simulink model "System"  (R2021b)
settings: Solver=VariableStepAuto  StartTime=0.0  StopTime=10  RelTol=1e-3
values from neighbouring files (symbols this model uses):
  a = 1.2    [new_ref1.mat]
  Cf = 19000    [new_ref1.mat]
  Iz = 3344    [new_ref1.mat]
  m = 2050    [new_ref1.mat]
libraries: simulink x1, mpclib x1
settings Model: Creator=gaura  LastModifiedBy=gaura

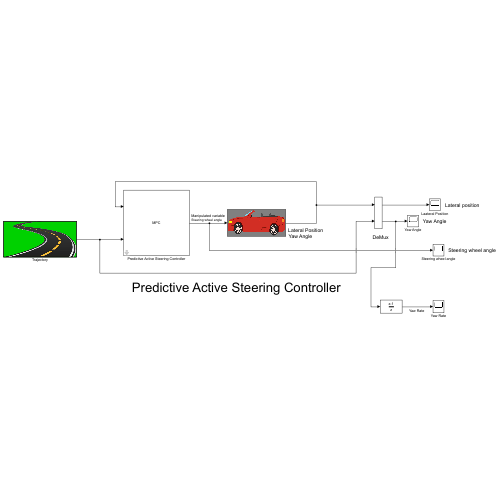
[thumbnail: Simulink's stored preview of the top-level diagram]
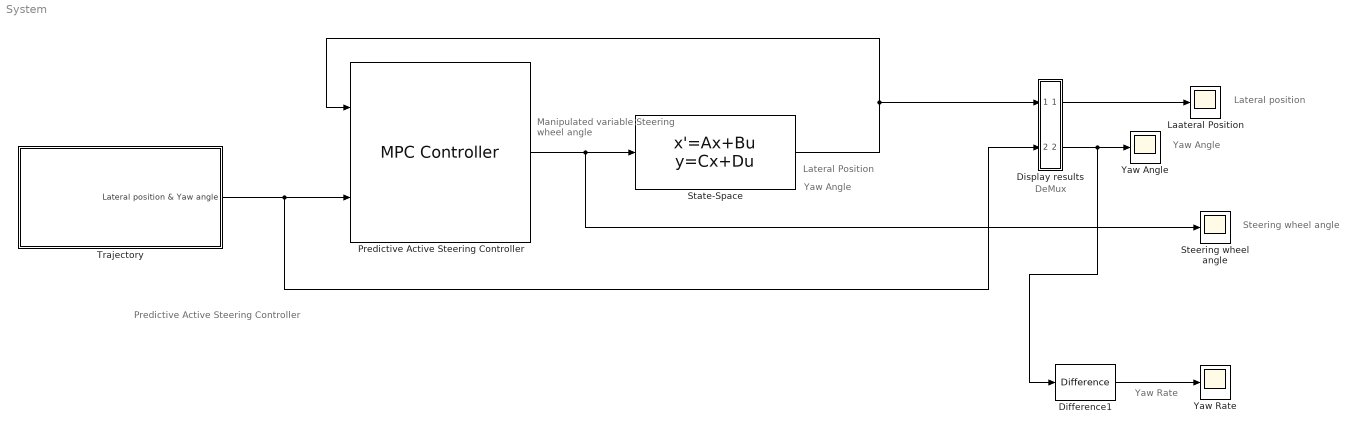
== system System ==
  note: Yaw Rate
  note: Steering wheel angle
  note: Predictive Active Steering Controller
  note: DeMux
  note: Yaw Angle
  note: Lateral Position
  note: Yaw Angle
  note: Lateral position
  note: Manipulated variable
      | Steering wheel angle
  Difference1 : simulink/Discrete/Difference  ICPrevInput=0.0  OutMin=[]  OutMax=[]  OutDataType=fixdt(1, 16)  OutScaling=2^-10  DoSatur=off
  Display results : Subsystem
  Laateral Position : Scope
  Predictive Active Steering Controller : mpclib/MPC Controller  SCDEnableBlockLinearizationSpecification=on  mpcobj=mpc1  is_multiple=0  enable_value=0  return_u0=off  updateMPCinCallerWorkspace=on  md_inport=off  mv_inport=off  uref_inport=off  return_cost=off  return_mvseq=off  return_qpstatus=off  return_xseq=off  return_state=off  return_ovseq=off  state_inport=off  umin_inport=off  umax_inport=off  ymin_inport=off  ymax_inport=off  cc_inport=off  ywt_inport=off  uwt_inport=off  duwt_inport=off  rhoeps_inport=off  pm_inport=off  MaximumP=10  HorizonChoice=FixedHorizon  n_ts=0.05  n_p=7  n_mv=1  n_md=0  n_ud=0  n_mo=2  n_uo=0  BlockDataType=double  SampleTimeInherited=off  switch_inport=off  mask(MPC){}
      mask Display:
      | % This is a new mask on top of the base mask.
      | % Use "View base mask" link below to see the base mask.
      | fprintf('MPC');
  State-Space : StateSpace  A=|  B=[2*Cf/m 0 2*Cf*a/Iz 0]'  C=[0 0 0 1;0 1 0 0]  D=[0;0]  InitialCondition=0
      | [-(2*Cf+2*Cr)/m/Vx, 0, -Vx-(2*Cf*a-2*Cr*b)/m/Vx, 0;
      |      0, 0, 1, 0;
      |      -(2*Cf*a-2*Cr*b)/Iz/Vx, 0, -(2*Cf*a^2+2*Cr*b^2)/Iz/Vx, 0;
      |      1, Vx, 0, 0]
      mask Display: image('convertible-car-png.png'); % Use "Edit Image" on toolstrip to change.
  Steering wheel angle : Scope
  Trajectory : Subsystem  TreatAsAtomicUnit=on
      mask Display: image('road_PNG48.png'); % Use "Edit Image" on toolstrip to change.
  Yaw Angle : Scope
  Yaw Rate : Scope
  wires:
  Predictive Active Steering Controller/1 -> Steering wheel angle/1, State-Space/1
  State-Space/1 -> Predictive Active Steering Controller/1, Display results/1(Outputs)
  Trajectory/1(Lateral position & Yaw angle) -> Display results/2(References), Predictive Active Steering Controller/2
  Display results/1(Out2) -> Laateral Position/1
  Display results/2(Out1) -> Difference1/1, Yaw Angle/1
  Difference1/1 -> Yaw Rate/1

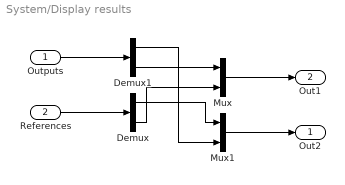
== system System/Display results ==
  Outputs : Inport
  References : Inport  Port=2
  Demux : Demux  Outputs=2
  Demux1 : Demux  Outputs=2
  Mux : Mux  Inputs=2
  Mux1 : Mux  Inputs=2
  Out2 : Outport  VectorParamsAs1DForOutWhenUnconnected=off
  Out1 : Outport  Port=2  VectorParamsAs1DForOutWhenUnconnected=off
  wires:
  References/1 -> Demux/1
  Outputs/1 -> Demux1/1
  Mux1/1 -> Out2/1
  Demux1/2 -> Mux/1
  Demux/1 -> Mux1/1
  Demux1/1 -> Mux1/2
  Mux/1 -> Out1/1
  Demux/2 -> Mux/2

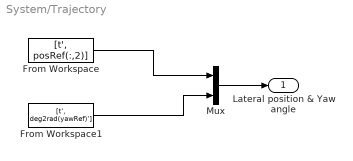
== system System/Trajectory ==
  From Workspace : FromWorkspace  VariableName=[t', posRef(:,2)]  SampleTime=0.1
  From Workspace1 : FromWorkspace  VariableName=[t', deg2rad(yawRef)']  SampleTime=0.1
  Mux : Mux  Inputs=2
  Lateral position & Yaw angle : Outport  VectorParamsAs1DForOutWhenUnconnected=off
  wires:
  Mux/1 -> Lateral position & Yaw angle/1
  From Workspace1/1 -> Mux/2
  From Workspace/1 -> Mux/1
